simulink model "untitled"  (Simulink 5.1)
settings: Solver=ode45  StartTime=0.0  StopTime=10.0  RelTol=1e-3
settings Model: LastModifiedBy=Administrator  BooleanDataType=on  ProdHWDeviceType=Microprocessor

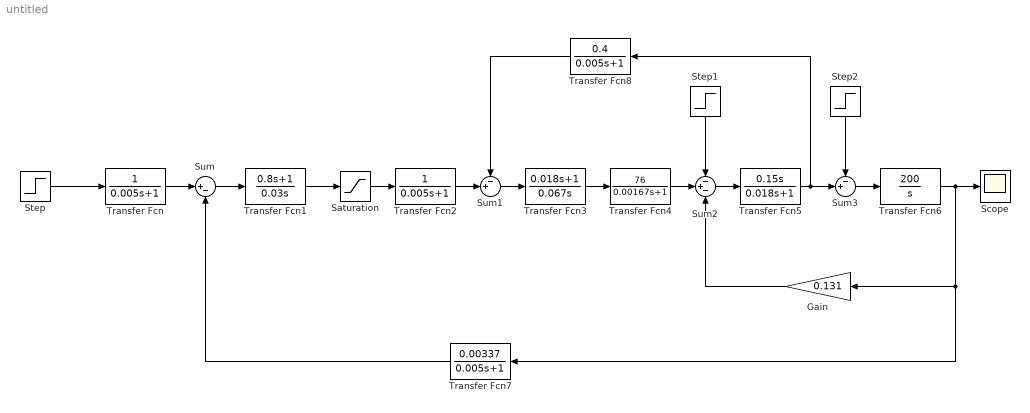
== system untitled ==
  Gain : Gain  Orientation=left  Gain=0.131  SaturateOnIntegerOverflow=on
  Saturation : Saturate  UpperLimit=8  LowerLimit=-8
  Scope : Scope
  Step : Step  After=10  SampleTime=0
  Step1 : Step  Orientation=down  Time=6  After=15  SampleTime=0
  Step2 : Step  Orientation=down  Time=8  After=15  SampleTime=0
  Sum : Sum  Inputs=|+-  SaturateOnIntegerOverflow=on
  Sum1 : Sum  Inputs=-+|  SaturateOnIntegerOverflow=on
  Sum2 : Sum  Inputs=-+-  SaturateOnIntegerOverflow=on
  Sum3 : Sum  Inputs=-+|  SaturateOnIntegerOverflow=on
  Transfer Fcn : TransferFcn  Denominator=[0.005 1]
  Transfer Fcn1 : TransferFcn  Numerator=[0.8 1]  Denominator=[0.03 0]
  Transfer Fcn2 : TransferFcn  Denominator=[0.005 1]
  Transfer Fcn3 : TransferFcn  Numerator=[0.018 1]  Denominator=[0.067 0]
  Transfer Fcn4 : TransferFcn  Numerator=[76]  Denominator=[0.00167 1]
  Transfer Fcn5 : TransferFcn  Numerator=[0.15 0]  Denominator=[0.018 1]
  Transfer Fcn6 : TransferFcn  Numerator=[200]  Denominator=[1 0]
  Transfer Fcn7 : TransferFcn  Orientation=left  Numerator=[0.00337]  Denominator=[0.005 1]
  Transfer Fcn8 : TransferFcn  Orientation=left  Numerator=[0.4]  Denominator=[0.005 1]
  wires:
  Step/1 -> Transfer Fcn/1
  Transfer Fcn/1 -> Sum/1
  Sum/1 -> Transfer Fcn1/1
  Transfer Fcn1/1 -> Saturation/1
  Saturation/1 -> Transfer Fcn2/1
  Sum1/1 -> Transfer Fcn3/1
  Transfer Fcn3/1 -> Transfer Fcn4/1
  Sum2/1 -> Transfer Fcn5/1
  Transfer Fcn6/1 -> Scope/1, Transfer Fcn7/1, Gain/1
  Transfer Fcn7/1 -> Sum/2
  Transfer Fcn2/1 -> Sum1/2
  Transfer Fcn5/1 -> Sum3/2, Transfer Fcn8/1
  Sum3/1 -> Transfer Fcn6/1
  Transfer Fcn8/1 -> Sum1/1
  Transfer Fcn4/1 -> Sum2/2
  Gain/1 -> Sum2/3
  Step1/1 -> Sum2/1
  Step2/1 -> Sum3/1
